simulink model "model_sine_unsaturated"  (R2024b)
settings: Solver=VariableStepAuto  StartTime=0.0  StopTime=10.0  RelTol=1e-3
values from neighbouring files (symbols this model uses):
  denC = denCA    [carson.m]
  denG = G.Denominator{1}    [carson.m]
  numC = numCA    [carson.m]
  numG = G.Numerator{1}    [carson.m]
  w_in = w_in_set(i)    [carson.m]
settings Model: Creator=carso  LastModifiedBy=carso

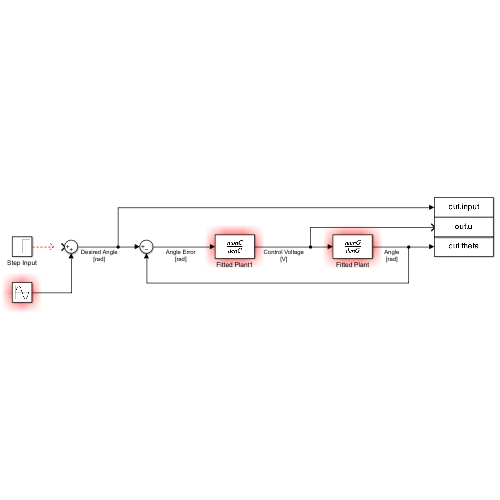
[thumbnail: Simulink's stored preview of the top-level diagram]
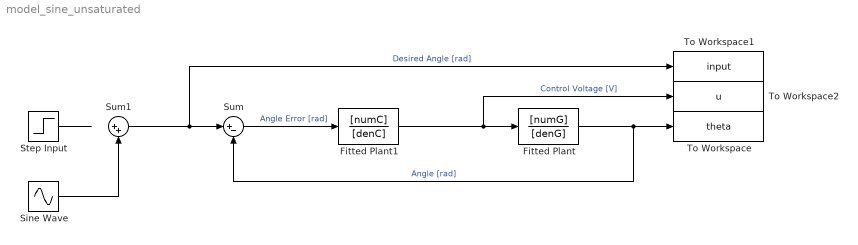
== system model_sine_unsaturated ==
  Fitted Plant : TransferFcn  Numerator=[numG]  Denominator=[denG]
  Fitted Plant1 : TransferFcn  Numerator=[numC]  Denominator=[denC]
  Sine Wave : Sin  Amplitude=0.5  Frequency=w_in  SampleTime=0
  Step Input : Step  SampleTime=0
  Sum : Sum  Inputs=|+-
  Sum1 : Sum  Inputs=|++
  To Workspace : ToWorkspace  VariableName=theta  SaveFormat=Timeseries  SampleTime=-1
  To Workspace1 : ToWorkspace  VariableName=input  SaveFormat=Timeseries  SampleTime=-1
  To Workspace2 : ToWorkspace  VariableName=u  SaveFormat=Timeseries  SampleTime=-1
  wires:
  Sum/1 -> Fitted Plant1/1  "Angle Error [rad]"
  Fitted Plant/1 -> Sum/2, To Workspace/1  "Angle [rad]"
  Step Input/1 -> ?
  Sine Wave/1 -> Sum1/2
  Sum1/1 -> To Workspace1/1, Sum/1  "Desired Angle [rad]"
  Fitted Plant1/1 -> To Workspace2/1, Fitted Plant/1  "Control Voltage [V]"
